simulink model "satellite_ADCS_slew_simulation"  (R2022b)
settings: Solver=FixedStepAuto  StartTime=t0  StopTime=t0+dt_po  FixedStep=0.1  RelTol=1e-9  AbsTol=1e-9
values from neighbouring files (symbols this model uses):
  A0 = Af    [satellite_ADCS_LEOP_simulation.m]
  A_sb_1 = [999.999999992226e-003    3.46376307675883e-006   -1.88420189887425e-006 ... (first row only)    [satellite_ADCS_LEOP_simulation.m]
  A_sb_2 = [999.999999948501e-003   -10.1488410044293e-006   -22.0178875132149e-012 ... (first row only)    [satellite_ADCS_LEOP_simulation.m]
  A_sb_3 = [999.999999975613e-003   -46.6812699606578e-012    6.98384920637069e-006 ... (first row only)    [satellite_ADCS_LEOP_simulation.m]
  alphaG_0 = pi/1.5    (= 2.09439510239)    [satellite_ADCS_LEOP_simulation.m]
  E = 1    [satellite_ADCS_LEOP_simulation.m]
  F = 1e-3    (= 0.001)    [satellite_ADCS_LEOP_simulation.m]
  FOV = deg2rad(21.7)    [satellite_ADCS_LEOP_simulation.m]
  g_nm = S_matrix.*g_coefficients    [satellite_ADCS_LEOP_simulation.m]
  h_nm = S_matrix.*h_coefficients    [satellite_ADCS_LEOP_simulation.m]
  J = diag([Ix,Iy,Iz])    [satellite_ADCS_LEOP_simulation.m]
  J2 = 1.082e-3    (= 0.001082)    [satellite_ADCS_LEOP_simulation.m]
  K_matrix = zeros(5,6)    [satellite_ADCS_LEOP_simulation.m]
  kdx = 0.001*450/8    (= 0.05625)    [satellite_ADCS_LEOP_simulation.m]
  kdy = kdx    (= 0.05625)    [satellite_ADCS_LEOP_simulation.m]
  kdz = kdy    (= 0.05625)    [satellite_ADCS_LEOP_simulation.m]
  kep = [a e i OM om thf]    [satellite_ADCS_LEOP_simulation.m]
  kpx = 0.6*0.001    (= 0.0006)    [satellite_ADCS_LEOP_simulation.m]
  kpy = kpx    (= 0.0006)    [satellite_ADCS_LEOP_simulation.m]
  kpz = kpy    (= 0.0006)    [satellite_ADCS_LEOP_simulation.m]
  LL = 1e-5    (= 1e-05)    [satellite_ADCS_LEOP_simulation.m]
  m = [0.37 0.32 0.28]    [satellite_ADCS_LEOP_simulation.m]
  mu = astroConstants(13)    [satellite_ADCS_LEOP_simulation.m]
  n_sun = 2*pi/T_y    (= 1.99238499086e-07)    [satellite_ADCS_LEOP_simulation.m]
  omega_e = 2*pi/T_e    (= 7.27220521664e-05)    [satellite_ADCS_LEOP_simulation.m]
  P00 = 1    [satellite_ADCS_LEOP_simulation.m]
  pR = pinv(R)    [satellite_ADCS_LEOP_simulation.m]
  R = [0 0 dz/2 0 0 -dz/2 ... (first row only)    [satellite_ADCS_LEOP_simulation.m]
  rt = astroConstants(23)    [satellite_ADCS_LEOP_simulation.m]
  S = S'    [satellite_ADCS_LEOP_simulation.m]
  sensor_noise = deg2rad(50/3600)    [satellite_ADCS_LEOP_simulation.m]
  sensor_sample_time = 1    [satellite_ADCS_LEOP_simulation.m]
  t0 = tf    (= 3200)    [satellite_ADCS_LEOP_simulation.m]
  T_o = 2*pi/n    [satellite_ADCS_LEOP_simulation.m]
  Te = 0.03    [satellite_ADCS_LEOP_simulation.m]
  Tp = [999.999926226686e-003    355.891478141766e-006   -144.526391847740e-006 ... (first row only)    [satellite_ADCS_LEOP_simulation.m]
  UL = 1e-4    (= 0.0001)    [satellite_ADCS_LEOP_simulation.m]
  w0 = wf    [satellite_ADCS_LEOP_simulation.m]
libraries: matrix_library x7, vrlib x3, slpidlib x3, sharedutil x2, aerolibutil x2
(part 3 of 3)

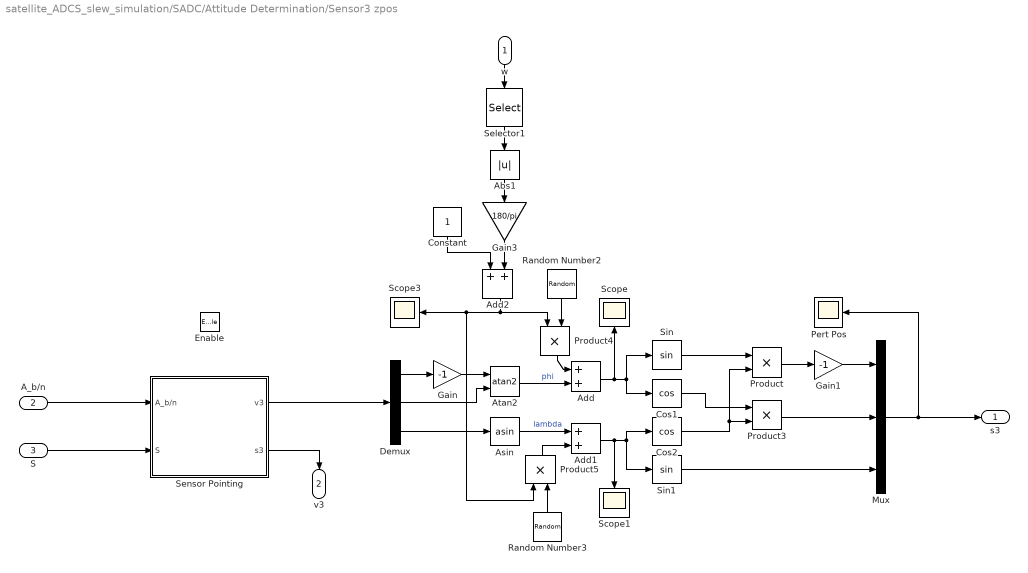
== system satellite_ADCS_slew_simulation/SADC/Attitude Determination/Sensor3 zpos ==
  w : Inport
  A_b/n : Inport  Port=2
  S : Inport  Port=3
  Enable : EnablePort  PropagateVarSize=During execution
  Abs1 : Abs  SaturateOnIntegerOverflow=off
  Add : Sum
  Add1 : Sum
  Add2 : Sum
  Asin : Trigonometry  Operator=asin
  Atan2 : Trigonometry  Operator=atan2
  Constant : Constant
  Cos1 : Trigonometry  Operator=cos
  Cos2 : Trigonometry  Operator=cos
  Demux : Demux  Outputs=3
  Gain : Gain  Gain=-1
  Gain1 : Gain  Gain=-1
  Gain3 : Gain  Gain=180/pi
  Mux : Mux  Inputs=3
  Pert Pos : Scope
  Product{,3..5} (4 alike) : Product
  Random Number2 : RandomNumber  Variance=sensor_noise^2  SampleTime=sensor_sample_time
  Random Number3 : RandomNumber  Variance=sensor_noise^2  SampleTime=sensor_sample_time
  Scope : Scope
  Scope1 : Scope
  Scope3 : Scope
  Selector1 : Selector  InputPortWidth=3  IndexOptions=Index vector (dialog)  Indices=3  OutputSizes=1
  Sensor Pointing : Subsystem
  Sin : Trigonometry
  Sin1 : Trigonometry
  s3 : Outport
  v3 : Outport  Port=2
  wires:
  Sensor Pointing/2(s3) -> v3/1
  Sensor Pointing/1(v3) -> Demux/1
  S/1 -> Sensor Pointing/2(S)
  A_b/n/1 -> Sensor Pointing/1(A_b/n)
  Gain1/1 -> Mux/1
  Sin1/1 -> Mux/3
  Mux/1 -> Pert Pos/1, s3/1
  Demux/3 -> Asin/1
  Product3/1 -> Mux/2
  Cos1/1 -> Product3/1
  Gain/1 -> Atan2/1
  Product/1 -> Gain1/1
  Sin/1 -> Product/1
  Add1/1 -> Cos2/1, Sin1/1, Scope1/1
  Cos2/1 -> Product3/2, Product/2
  Atan2/1 -> Add/2  "phi"
  Asin/1 -> Add1/1  "lambda"
  Demux/2 -> Atan2/2
  Add/1 -> Scope/1, Sin/1, Cos1/1
  Demux/1 -> Gain/1
  Product4/1 -> Add/1
  Product5/1 -> Add1/2
  w/1 -> Selector1/1
  Random Number2/1 -> Product4/2
  Add2/1 -> Product4/1, Scope3/1, Product5/1
  Selector1/1 -> Abs1/1
  Random Number3/1 -> Product5/2
  Abs1/1 -> Gain3/1
  Constant/1 -> Add2/1
  Gain3/1 -> Add2/2

== system satellite_ADCS_slew_simulation/SADC/Attitude Determination/Sun Sensors ==
  S_n : Inport
  A_b/n : Inport  Port=2
  Mux : Mux  Inputs=3
  Sun Sensor xpos : Subsystem
  Sun Sensor ypos : Subsystem
  Sun Sensor zpos : Subsystem
  Sun Obstruction : Outport
  wires:
  Mux/1 -> Sun Obstruction/1
  Sun Sensor zpos/1(s3) -> Mux/3
  Sun Sensor xpos/1(s1) -> Mux/1
  Sun Sensor ypos/1(s2) -> Mux/2
  S_n/1 -> Sun Sensor ypos/2(S_n), Sun Sensor zpos/2(S_n), Sun Sensor xpos/2(S_n)
  A_b/n/1 -> Sun Sensor ypos/1(A_b/n), Sun Sensor zpos/1(A_b/n), Sun Sensor xpos/1(A_b/n)

== system satellite_ADCS_slew_simulation/SADC/Attitude Determination/Wabha Attitude Determination ==
  s1 : Inport
  v1 : Inport  Port=2
  s2 : Inport  Port=3
  v2 : Inport  Port=4
  s3 : Inport  Port=5
  v3 : Inport  Port=6
  E : Inport  Port=7
  If : If  IfExpression=u1 == 3
  Merge : Merge
  Scope : Scope
  Sum of Elements : Sum  Inputs=+
  Wabha Attitude Determination 2s : Subsystem
  Wabha Attitude Determination 3s : Subsystem
  A*_b/n : Outport
  wires:
  v3/1 -> Wabha Attitude Determination 2s/7(v3), Wabha Attitude Determination 3s/6(v3)
  s3/1 -> Wabha Attitude Determination 2s/6(s3), Wabha Attitude Determination 3s/5(s3)
  v2/1 -> Wabha Attitude Determination 2s/5(v2), Wabha Attitude Determination 3s/4(v2)
  s2/1 -> Wabha Attitude Determination 2s/4(s2), Wabha Attitude Determination 3s/3(s2)
  v1/1 -> Wabha Attitude Determination 2s/3(v1), Wabha Attitude Determination 3s/2(v1)
  s1/1 -> Wabha Attitude Determination 2s/2(s1), Wabha Attitude Determination 3s/1(s1)
  Merge/1 -> A*_b/n/1
  If/1 -> Wabha Attitude Determination 3s/Action
  Wabha Attitude Determination 2s/1(A*_b/n) -> Merge/1
  If/2 -> Wabha Attitude Determination 2s/Action
  E/1 -> Sum of Elements/1, Wabha Attitude Determination 2s/1(E)
  Wabha Attitude Determination 3s/1(A*_b/n) -> Merge/2
  Sum of Elements/1 -> If/1, Scope/1

== system satellite_ADCS_slew_simulation/Euler Angles Kinematics/312 kin/R312/R1 ==
  a : Inport
  Add : Sum  Inputs=+++
  Constant : Constant  Value=[0 0 0; 0 1 0; 0 0 1]
  Constant1 : Constant  Value=[0 0 0; 0 0 -1; 0 1 0]
  Constant2 : Constant  Value=[1 0 0; 0 0 0; 0 0 0]
  Cos : Trigonometry  Operator=cos
  Product : Product
  Product1 : Product
  Sin : Trigonometry
  R1 : Outport
  wires:
  a/1 -> Cos/1, Sin/1
  Cos/1 -> Product/2
  Constant/1 -> Product/1
  Constant1/1 -> Product1/1
  Sin/1 -> Product1/2
  Product/1 -> Add/1
  Constant2/1 -> Add/3
  Product1/1 -> Add/2
  Add/1 -> R1/1

== system satellite_ADCS_slew_simulation/Euler Angles Kinematics/312 kin/R312/R2 ==
  a : Inport
  Add : Sum  Inputs=+++
  Constant : Constant  Value=[1 0 0; 0 0 0; 0 0 1]
  Constant1 : Constant  Value=[0 0 1; 0 0 0; -1 0 0]
  Constant2 : Constant  Value=[0 0 0; 0 1 0; 0 0 0]
  Cos : Trigonometry  Operator=cos
  Product : Product
  Product1 : Product
  Sin : Trigonometry
  R2 : Outport
  wires:
  a/1 -> Cos/1, Sin/1
  Cos/1 -> Product/2
  Constant/1 -> Product/1
  Constant1/1 -> Product1/1
  Sin/1 -> Product1/2
  Product/1 -> Add/1
  Constant2/1 -> Add/3
  Product1/1 -> Add/2
  Add/1 -> R2/1

== system satellite_ADCS_slew_simulation/Euler Angles Kinematics/312 kin/R312/R3 ==
  a : Inport
  Add : Sum  Inputs=+++
  Constant : Constant  Value=[1 0 0; 0 1 0; 0 0 0]
  Constant1 : Constant  Value=[0 -1 0; 1 0 0; 0 0 0]
  Constant2 : Constant  Value=[0 0 0; 0 0 0; 0 0 1]
  Cos : Trigonometry  Operator=cos
  Product : Product
  Product1 : Product
  Sin : Trigonometry
  R3 : Outport
  wires:
  a/1 -> Cos/1, Sin/1
  Cos/1 -> Product/2
  Constant/1 -> Product/1
  Constant1/1 -> Product1/1
  Sin/1 -> Product1/2
  Product/1 -> Add/1
  Constant2/1 -> Add/3
  Product1/1 -> Add/2
  Add/1 -> R3/1

== system satellite_ADCS_slew_simulation/Euler Angles Kinematics/312 kin/R313/R1 ==
  a : Inport
  Add : Sum  Inputs=+++
  Constant : Constant  Value=[0 0 0; 0 1 0; 0 0 1]
  Constant1 : Constant  Value=[0 0 0; 0 0 -1; 0 1 0]
  Constant2 : Constant  Value=[1 0 0; 0 0 0; 0 0 0]
  Cos : Trigonometry  Operator=cos
  Product : Product
  Product1 : Product
  Sin : Trigonometry
  R1 : Outport
  wires:
  a/1 -> Cos/1, Sin/1
  Cos/1 -> Product/2
  Constant/1 -> Product/1
  Constant1/1 -> Product1/1
  Sin/1 -> Product1/2
  Product/1 -> Add/1
  Constant2/1 -> Add/3
  Product1/1 -> Add/2
  Add/1 -> R1/1

== system satellite_ADCS_slew_simulation/Euler Angles Kinematics/312 kin/R313/R3 ==
  a : Inport
  Add : Sum  Inputs=+++
  Constant : Constant  Value=[1 0 0; 0 1 0; 0 0 0]
  Constant1 : Constant  Value=[0 -1 0; 1 0 0; 0 0 0]
  Constant2 : Constant  Value=[0 0 0; 0 0 0; 0 0 1]
  Cos : Trigonometry  Operator=cos
  Product : Product
  Product1 : Product
  Sin : Trigonometry
  R3 : Outport
  wires:
  a/1 -> Cos/1, Sin/1
  Cos/1 -> Product/2
  Constant/1 -> Product/1
  Constant1/1 -> Product1/1
  Sin/1 -> Product1/2
  Product/1 -> Add/1
  Constant2/1 -> Add/3
  Product1/1 -> Add/2
  Add/1 -> R3/1

== system satellite_ADCS_slew_simulation/Euler Angles Kinematics/312 kin/R313/R3' ==
  a : Inport
  Add : Sum  Inputs=+++
  Constant : Constant  Value=[1 0 0; 0 1 0; 0 0 0]
  Constant1 : Constant  Value=[0 -1 0; 1 0 0; 0 0 0]
  Constant2 : Constant  Value=[0 0 0; 0 0 0; 0 0 1]
  Cos : Trigonometry  Operator=cos
  Product : Product
  Product1 : Product
  Sin : Trigonometry
  R3 : Outport
  wires:
  a/1 -> Cos/1, Sin/1
  Cos/1 -> Product/2
  Constant/1 -> Product/1
  Constant1/1 -> Product1/1
  Sin/1 -> Product1/2
  Product/1 -> Add/1
  Constant2/1 -> Add/3
  Product1/1 -> Add/2
  Add/1 -> R3/1

== system satellite_ADCS_slew_simulation/Euler Angles Kinematics/313 kin/R312/R1 ==
  a : Inport
  Add : Sum  Inputs=+++
  Constant : Constant  Value=[0 0 0; 0 1 0; 0 0 1]
  Constant1 : Constant  Value=[0 0 0; 0 0 -1; 0 1 0]
  Constant2 : Constant  Value=[1 0 0; 0 0 0; 0 0 0]
  Cos : Trigonometry  Operator=cos
  Product : Product
  Product1 : Product
  Sin : Trigonometry
  R1 : Outport
  wires:
  a/1 -> Cos/1, Sin/1
  Cos/1 -> Product/2
  Constant/1 -> Product/1
  Constant1/1 -> Product1/1
  Sin/1 -> Product1/2
  Product/1 -> Add/1
  Constant2/1 -> Add/3
  Product1/1 -> Add/2
  Add/1 -> R1/1

== system satellite_ADCS_slew_simulation/Euler Angles Kinematics/313 kin/R312/R2 ==
  a : Inport
  Add : Sum  Inputs=+++
  Constant : Constant  Value=[1 0 0; 0 0 0; 0 0 1]
  Constant1 : Constant  Value=[0 0 1; 0 0 0; -1 0 0]
  Constant2 : Constant  Value=[0 0 0; 0 1 0; 0 0 0]
  Cos : Trigonometry  Operator=cos
  Product : Product
  Product1 : Product
  Sin : Trigonometry
  R2 : Outport
  wires:
  a/1 -> Cos/1, Sin/1
  Cos/1 -> Product/2
  Constant/1 -> Product/1
  Constant1/1 -> Product1/1
  Sin/1 -> Product1/2
  Product/1 -> Add/1
  Constant2/1 -> Add/3
  Product1/1 -> Add/2
  Add/1 -> R2/1

== system satellite_ADCS_slew_simulation/Euler Angles Kinematics/313 kin/R312/R3 ==
  a : Inport
  Add : Sum  Inputs=+++
  Constant : Constant  Value=[1 0 0; 0 1 0; 0 0 0]
  Constant1 : Constant  Value=[0 -1 0; 1 0 0; 0 0 0]
  Constant2 : Constant  Value=[0 0 0; 0 0 0; 0 0 1]
  Cos : Trigonometry  Operator=cos
  Product : Product
  Product1 : Product
  Sin : Trigonometry
  R3 : Outport
  wires:
  a/1 -> Cos/1, Sin/1
  Cos/1 -> Product/2
  Constant/1 -> Product/1
  Constant1/1 -> Product1/1
  Sin/1 -> Product1/2
  Product/1 -> Add/1
  Constant2/1 -> Add/3
  Product1/1 -> Add/2
  Add/1 -> R3/1

== system satellite_ADCS_slew_simulation/Euler Angles Kinematics/313 kin/R313/R1 ==
  a : Inport
  Add : Sum  Inputs=+++
  Constant : Constant  Value=[0 0 0; 0 1 0; 0 0 1]
  Constant1 : Constant  Value=[0 0 0; 0 0 -1; 0 1 0]
  Constant2 : Constant  Value=[1 0 0; 0 0 0; 0 0 0]
  Cos : Trigonometry  Operator=cos
  Product : Product
  Product1 : Product
  Sin : Trigonometry
  R1 : Outport
  wires:
  a/1 -> Cos/1, Sin/1
  Cos/1 -> Product/2
  Constant/1 -> Product/1
  Constant1/1 -> Product1/1
  Sin/1 -> Product1/2
  Product/1 -> Add/1
  Constant2/1 -> Add/3
  Product1/1 -> Add/2
  Add/1 -> R1/1

== system satellite_ADCS_slew_simulation/Euler Angles Kinematics/313 kin/R313/R3 ==
  a : Inport
  Add : Sum  Inputs=+++
  Constant : Constant  Value=[1 0 0; 0 1 0; 0 0 0]
  Constant1 : Constant  Value=[0 -1 0; 1 0 0; 0 0 0]
  Constant2 : Constant  Value=[0 0 0; 0 0 0; 0 0 1]
  Cos : Trigonometry  Operator=cos
  Product : Product
  Product1 : Product
  Sin : Trigonometry
  R3 : Outport
  wires:
  a/1 -> Cos/1, Sin/1
  Cos/1 -> Product/2
  Constant/1 -> Product/1
  Constant1/1 -> Product1/1
  Sin/1 -> Product1/2
  Product/1 -> Add/1
  Constant2/1 -> Add/3
  Product1/1 -> Add/2
  Add/1 -> R3/1

== system satellite_ADCS_slew_simulation/Euler Angles Kinematics/313 kin/R313/R3' ==
  a : Inport
  Add : Sum  Inputs=+++
  Constant : Constant  Value=[1 0 0; 0 1 0; 0 0 0]
  Constant1 : Constant  Value=[0 -1 0; 1 0 0; 0 0 0]
  Constant2 : Constant  Value=[0 0 0; 0 0 0; 0 0 1]
  Cos : Trigonometry  Operator=cos
  Product : Product
  Product1 : Product
  Sin : Trigonometry
  R3 : Outport
  wires:
  a/1 -> Cos/1, Sin/1
  Cos/1 -> Product/2
  Constant/1 -> Product/1
  Constant1/1 -> Product1/1
  Sin/1 -> Product1/2
  Product/1 -> Add/1
  Constant2/1 -> Add/3
  Product1/1 -> Add/2
  Add/1 -> R3/1

== system satellite_ADCS_slew_simulation/SADC/Attitude Determination/Algebraic Attitude Determination/2s Method ==
  S : Inport
  V : Inport  Port=2
  E : Inport  Port=3
  Enable : EnablePort  PropagateVarSize=During execution
  Cross Product{,1..3} (4 alike) : matrix_library/Cross Product
  Find Nonzero Elements : Find  NumberOfInputDimensions=3
  Invert 3x3 Matrix : aerolibutil/Invert  3x3 Matrix
  MatrixMultiply : Product  Multiplication=Matrix(*)
  Normalize Vector : vrlib/Utilities/Normalize Vector  maxzero=0
  Normalize Vector1 : vrlib/Utilities/Normalize Vector  maxzero=0
  Selector : Selector  NumberOfDimensions=2  InputPortWidth=3  IndexOptions=Index vector (dialog),Index vector (dialog)  Indices=[1 2 3],1  OutputSizes=1,1
  Selector1 : Selector  NumberOfDimensions=2  InputPortWidth=3  IndexOptions=Index vector (dialog),Index vector (dialog)  Indices=[1 2 3],2  OutputSizes=1,1
  Selector2 : Selector  NumberOfDimensions=2  InputPortWidth=3  IndexOptions=Index vector (dialog),Index vector (dialog)  Indices=[1 2 3],1  OutputSizes=1,1
  Selector3 : Selector  NumberOfDimensions=2  InputPortWidth=3  IndexOptions=Index vector (dialog),Index vector (dialog)  Indices=[1 2 3],2  OutputSizes=1,1
  Selector4 : Selector  NumberOfDimensions=2  InputPortWidth=3  IndexOptions=Index vector (dialog),Index vector (port)  Indices=[1 2 3],1  OutputSizes=1,1
  Selector5 : Selector  NumberOfDimensions=2  InputPortWidth=3  IndexOptions=Index vector (dialog),Index vector (port)  Indices=[1 2 3],1  OutputSizes=1,1
  Vector Concatenate : Concatenate  NumInputs=3  Mode=Multidimensional array  ConcatenateDimension=2
  Vector Concatenate1 : Concatenate  NumInputs=3  Mode=Multidimensional array  ConcatenateDimension=2
  A_b/n : Outport
  wires:
  S/1 -> Selector5/1  "S"
  V/1 -> Selector4/1  "V"
  Find Nonzero Elements/1 -> Selector4/2, Selector5/2
  E/1 -> Find Nonzero Elements/1
  MatrixMultiply/1 -> A_b/n/1
  Invert 3x3 Matrix/1 -> MatrixMultiply/2
  Vector Concatenate1/1 -> Invert 3x3 Matrix/1  "V"
  Vector Concatenate/1 -> MatrixMultiply/1  "S"
  Cross Product3/1 -> Vector Concatenate1/3
  Cross Product2/1 -> Vector Concatenate/3
  Normalize Vector/1 -> Cross Product3/2, Vector Concatenate1/2
  Normalize Vector1/1 -> Cross Product2/2, Vector Concatenate/2
  Cross Product/1 -> Normalize Vector1/1
  Cross Product1/1 -> Normalize Vector/1
  Selector3/1 -> Cross Product1/2  "b"
  Selector2/1 -> Cross Product1/1, Vector Concatenate1/1, Cross Product3/1  "a"
  Selector1/1 -> Cross Product/2  "q"
  Selector/1 -> Cross Product2/1, Vector Concatenate/1, Cross Product/1  "p"
  Selector5/1 -> Selector/1, Selector1/1  "S"
  Selector4/1 -> Selector2/1, Selector3/1  "V"

== system satellite_ADCS_slew_simulation/SADC/Attitude Determination/Algebraic Attitude Determination/3s Method ==
  S : Inport
  V : Inport  Port=2
  Enable : EnablePort  PropagateVarSize=During execution
  Invert 3x3 Matrix1 : aerolibutil/Invert  3x3 Matrix
  MatrixMultiply3 : Product  Multiplication=Matrix(*)
  A_b/n : Outport
  wires:
  S/1 -> MatrixMultiply3/1  "S"
  Invert 3x3 Matrix1/1 -> MatrixMultiply3/2  "V*"
  MatrixMultiply3/1 -> A_b/n/1
  V/1 -> Invert 3x3 Matrix1/1  "V"

== system satellite_ADCS_slew_simulation/SADC/Attitude Determination/Sensor1 xpos/Sensor Pointing ==
  note: A_b/n is already discretized
  note: A_sb is relative to the sensor
  note: star catalogue in inertial frame
  A_b/n : Inport
  S : Inport  Port=2
  . : Product  Multiplication=Matrix(*)
  Constant2 : Constant  Value=A_sb_1
  Constant4 : Constant  Value=FOV/2
  Cos : Trigonometry  Operator=cos
  Find Nonzero Elements1 : Find  NumberOfInputDimensions=3
  Less Than1 : RelationalOperator  OutDataTypeStr=boolean  RndMeth=Simplest  InputSameDT=off
  MinMax2 : MinMax
  Product1 : Product  Multiplication=Matrix(*)
  Scope3 : Scope
  Selector1 : Selector  NumberOfDimensions=2  InputPortWidth=3  IndexOptions=Index vector (dialog),Index vector (port)  Indices=[1 2 3],1  OutputSizes=1,1
  Selector2 : Selector  NumberOfDimensions=2  InputPortWidth=3  IndexOptions=Index vector (dialog),Index vector (port)  Indices=[1 2 3],1  OutputSizes=1,1
  x : Selector  NumberOfDimensions=2  InputPortWidth=3  IndexOptions=Index vector (dialog),Index vector (dialog)  Indices=1,1:162  OutputSizes=1,1
  s1 : Outport
  v1 : Outport  Port=2
  wires:
  A_b/n/1 -> Product1/2
  Selector1/1 -> v1/1
  Less Than1/1 -> Find Nonzero Elements1/1
  Cos/1 -> Less Than1/2
  x/1 -> Less Than1/1
  Product1/1 -> ./1  "A_s/n"
  S/1 -> ./2, Selector1/1
  Find Nonzero Elements1/1 -> MinMax2/1
  Constant4/1 -> Cos/1
  ./1 -> x/1, Selector2/1
  Selector2/1 -> Scope3/1, s1/1
  Constant2/1 -> Product1/1
  MinMax2/1 -> Selector1/2, Selector2/2

== system satellite_ADCS_slew_simulation/SADC/Attitude Determination/Sensor2 ypos/Sensor Pointing ==
  note: star catalogue in inertial frame
  note: A_sb is relative to the sensor
  note: A_b/n is already discretized
  A_b/n : Inport
  S : Inport  Port=2
  . : Product  Multiplication=Matrix(*)
  Constant2 : Constant  Value=A_sb_2
  Constant4 : Constant  Value=FOV/2
  Cos : Trigonometry  Operator=cos
  Find Nonzero Elements1 : Find  NumberOfInputDimensions=3
  Less Than1 : RelationalOperator  OutDataTypeStr=boolean  RndMeth=Simplest  InputSameDT=off
  MinMax2 : MinMax
  Product1 : Product  Multiplication=Matrix(*)
  Scope3 : Scope
  Selector1 : Selector  NumberOfDimensions=2  InputPortWidth=3  IndexOptions=Index vector (dialog),Index vector (port)  Indices=[1 2 3],1  OutputSizes=1,1
  Selector2 : Selector  NumberOfDimensions=2  InputPortWidth=3  IndexOptions=Index vector (dialog),Index vector (port)  Indices=[1 2 3],1  OutputSizes=1,1
  y : Selector  NumberOfDimensions=2  InputPortWidth=3  IndexOptions=Index vector (dialog),Index vector (dialog)  Indices=2,1:162  OutputSizes=1,1
  s2 : Outport
  v2 : Outport  Port=2
  wires:
  A_b/n/1 -> Product1/2
  Selector1/1 -> v2/1
  S/1 -> Selector1/1, ./2
  ./1 -> Selector2/1, y/1
  Constant4/1 -> Cos/1
  y/1 -> Less Than1/1
  Product1/1 -> ./1  "A_s/n"
  Find Nonzero Elements1/1 -> MinMax2/1
  Cos/1 -> Less Than1/2
  Constant2/1 -> Product1/1
  MinMax2/1 -> Selector2/2, Selector1/2
  Selector2/1 -> Scope3/1, s2/1
  Less Than1/1 -> Find Nonzero Elements1/1

== system satellite_ADCS_slew_simulation/SADC/Attitude Determination/Sensor3 zpos/Sensor Pointing ==
  note: A_b/n is already discretized
  note: A_sb is relative to the sensor
  note: star catalogue in inertial frame
  A_b/n : Inport
  S : Inport  Port=2
  . : Product  Multiplication=Matrix(*)
  Constant2 : Constant  Value=A_sb_3
  Constant4 : Constant  Value=FOV/2
  Cos : Trigonometry  Operator=cos
  Find Nonzero Elements1 : Find  NumberOfInputDimensions=3
  Less Than1 : RelationalOperator  OutDataTypeStr=boolean  RndMeth=Simplest  InputSameDT=off
  MinMax2 : MinMax
  Product1 : Product  Multiplication=Matrix(*)
  Scope3 : Scope
  Selector1 : Selector  NumberOfDimensions=2  InputPortWidth=3  IndexOptions=Index vector (dialog),Index vector (port)  Indices=[1 2 3],1  OutputSizes=1,1
  Selector2 : Selector  NumberOfDimensions=2  InputPortWidth=3  IndexOptions=Index vector (dialog),Index vector (port)  Indices=[1 2 3],1  OutputSizes=1,1
  z : Selector  NumberOfDimensions=2  InputPortWidth=3  IndexOptions=Index vector (dialog),Index vector (dialog)  Indices=3,1:162  OutputSizes=1,1
  v3 : Outport
  s3 : Outport  Port=2
  wires:
  Selector1/1 -> s3/1
  Product1/1 -> ./1  "A_s/n"
  z/1 -> Less Than1/1
  A_b/n/1 -> Product1/2
  Constant2/1 -> Product1/1
  Cos/1 -> Less Than1/2
  Less Than1/1 -> Find Nonzero Elements1/1
  ./1 -> z/1, Selector2/1
  S/1 -> ./2, Selector1/1
  Selector2/1 -> Scope3/1, v3/1
  MinMax2/1 -> Selector1/2, Selector2/2
  Constant4/1 -> Cos/1
  Find Nonzero Elements1/1 -> MinMax2/1

== system satellite_ADCS_slew_simulation/SADC/Attitude Determination/Sun Sensors/Sun Sensor xpos ==
  note: A_sb is relative to the sensor
  A_b/n : Inport
  S_n : Inport  Port=2
  . : Product  Multiplication=Matrix(*)
  Constant2 : Constant  Value=A_sb_1
  Constant4 : Constant  Value=1.5*FOV/2
  Cos : Trigonometry  Operator=cos
  Less Than1 : RelationalOperator  Operator=<=  OutDataTypeStr=boolean  RndMeth=Simplest  InputSameDT=off
  Product1 : Product  Multiplication=Matrix(*)
  x : Selector  InputPortWidth=3  IndexOptions=Index vector (dialog)  Indices=1  OutputSizes=1
  s1 : Outport
  wires:
  A_b/n/1 -> Product1/2
  Cos/1 -> Less Than1/2
  x/1 -> Less Than1/1
  Product1/1 -> ./1  "A_s/n"
  S_n/1 -> ./2
  Constant4/1 -> Cos/1
  ./1 -> x/1
  Less Than1/1 -> s1/1
  Constant2/1 -> Product1/1

== system satellite_ADCS_slew_simulation/SADC/Attitude Determination/Sun Sensors/Sun Sensor ypos ==
  note: A_sb is relative to the sensor
  A_b/n : Inport
  S_n : Inport  Port=2
  . : Product  Multiplication=Matrix(*)
  Constant2 : Constant  Value=A_sb_2
  Constant4 : Constant  Value=1.5*FOV/2
  Cos : Trigonometry  Operator=cos
  Less Than1 : RelationalOperator  Operator=<=  OutDataTypeStr=boolean  RndMeth=Simplest  InputSameDT=off
  Product1 : Product  Multiplication=Matrix(*)
  y : Selector  InputPortWidth=3  IndexOptions=Index vector (dialog)  Indices=2  OutputSizes=1
  s2 : Outport
  wires:
  A_b/n/1 -> Product1/2
  S_n/1 -> ./2
  ./1 -> y/1
  Constant4/1 -> Cos/1
  y/1 -> Less Than1/1
  Product1/1 -> ./1  "A_s/n"
  Cos/1 -> Less Than1/2
  Constant2/1 -> Product1/1
  Less Than1/1 -> s2/1

== system satellite_ADCS_slew_simulation/SADC/Attitude Determination/Sun Sensors/Sun Sensor zpos ==
  note: A_sb is relative to the sensor
  A_b/n : Inport
  S_n : Inport  Port=2
  . : Product  Multiplication=Matrix(*)
  Constant2 : Constant  Value=A_sb_3
  Constant4 : Constant  Value=1.5*FOV/2
  Cos : Trigonometry  Operator=cos
  Less Than1 : RelationalOperator  Operator=<=  OutDataTypeStr=boolean  RndMeth=Simplest  InputSameDT=off
  Product1 : Product  Multiplication=Matrix(*)
  z : Selector  InputPortWidth=3  IndexOptions=Index vector (dialog)  Indices=3  OutputSizes=1
  s3 : Outport
  wires:
  Product1/1 -> ./1  "A_s/n"
  z/1 -> Less Than1/1
  A_b/n/1 -> Product1/2
  Constant2/1 -> Product1/1
  Cos/1 -> Less Than1/2
  Less Than1/1 -> s3/1
  ./1 -> z/1
  S_n/1 -> ./2
  Constant4/1 -> Cos/1

== system satellite_ADCS_slew_simulation/SADC/Attitude Determination/Wabha Attitude Determination/Wabha Attitude Determination 2s ==
  E : Inport
  s1 : Inport  Port=2
  v1 : Inport  Port=3
  s2 : Inport  Port=4
  v2 : Inport  Port=5
  s3 : Inport  Port=6
  v3 : Inport  Port=7
  Action Port : ActionPort  PropagateVarSize=During execution  ActionPortLabel=else
  Add : Sum
  Constant3 : Constant  Value=1/2
  Find Nonzero Elements : Find  NumberOfInputDimensions=3
  MATLAB Function : MATLAB Function  TreatAsAtomicUnit=on
  Product : Product
  Product1 : Product
  Product3 : Product  Multiplication=Matrix(*)
  Product4 : Product  Multiplication=Matrix(*)
  Selector : Selector  NumberOfDimensions=2  InputPortWidth=3  IndexOptions=Index vector (dialog),Index vector (port)  Indices=[1 2 3],1  OutputSizes=1,1
  Selector1 : Selector  NumberOfDimensions=2  InputPortWidth=3  IndexOptions=Index vector (dialog),Index vector (port)  Indices=[1 2 3],1  OutputSizes=1,1
  Selector2 : Selector  NumberOfDimensions=2  InputPortWidth=3  IndexOptions=Index vector (dialog),Index vector (dialog)  Indices=[1 2 3],1  OutputSizes=1,1
  Selector3 : Selector  NumberOfDimensions=2  InputPortWidth=3  IndexOptions=Index vector (dialog),Index vector (dialog)  Indices=[1 2 3],2  OutputSizes=1,1
  Selector4 : Selector  NumberOfDimensions=2  InputPortWidth=3  IndexOptions=Index vector (dialog),Index vector (dialog)  Indices=[1 2 3],1  OutputSizes=1,1
  Selector5 : Selector  NumberOfDimensions=2  InputPortWidth=3  IndexOptions=Index vector (dialog),Index vector (dialog)  Indices=[1 2 3],2  OutputSizes=1,1
  Transpose : Math  Operator=transpose
  Transpose1 : Math  Operator=transpose
  Vector Concatenate : Concatenate  NumInputs=3  Mode=Multidimensional array  ConcatenateDimension=2
  Vector Concatenate1 : Concatenate  NumInputs=3  Mode=Multidimensional array  ConcatenateDimension=2
  A*_b/n : Outport
  wires:
  Constant3/1 -> Product/2, Product1/2
  MATLAB Function/1(y) -> A*_b/n/1
  Product1/1 -> Add/2
  Product/1 -> Add/1
  Transpose1/1 -> Product4/2
  Transpose/1 -> Product3/2
  Selector5/1 -> Transpose1/1  "v2"
  Selector4/1 -> Transpose/1  "v1"
  Selector3/1 -> Product4/1  "s2"
  Selector2/1 -> Product3/1  "s1"
  Product4/1 -> Product1/1
  Product3/1 -> Product/1
  Add/1 -> MATLAB Function/1(u)
  Selector/1 -> Selector5/1, Selector4/1
  Selector1/1 -> Selector2/1, Selector3/1
  Find Nonzero Elements/1 -> Selector1/2, Selector/2
  Vector Concatenate/1 -> Selector1/1
  Vector Concatenate1/1 -> Selector/1
  E/1 -> Find Nonzero Elements/1
  v1/1 -> Vector Concatenate1/1
  v2/1 -> Vector Concatenate1/2
  v3/1 -> Vector Concatenate1/3
  s3/1 -> Vector Concatenate/3
  s2/1 -> Vector Concatenate/2
  s1/1 -> Vector Concatenate/1

== system satellite_ADCS_slew_simulation/SADC/Attitude Determination/Wabha Attitude Determination/Wabha Attitude Determination 3s ==
  s1 : Inport
  v1 : Inport  Port=2
  s2 : Inport  Port=3
  v2 : Inport  Port=4
  s3 : Inport  Port=5
  v3 : Inport  Port=6
  Action Port : ActionPort  PropagateVarSize=During execution  ActionPortLabel=if(u1 == 3)
  Constant3 : Constant  Value=1/3
  MATLAB Function : MATLAB Function  TreatAsAtomicUnit=on
  Product : Product  Multiplication=Matrix(*)
  Product1 : Product  Multiplication=Matrix(*)
  Product2 : Product  Multiplication=Matrix(*)
  Product3 : Product
  Product4 : Product
  Product5 : Product
  Sum : Sum  Inputs=+++
  Transpose : Math  Operator=transpose
  Transpose1 : Math  Operator=transpose
  Transpose2 : Math  Operator=transpose
  A*_b/n : Outport
  wires:
  Constant3/1 -> Product5/2, Product4/2, Product3/2
  Sum/1 -> MATLAB Function/1(u)  "B"
  MATLAB Function/1(y) -> A*_b/n/1
  v1/1 -> Transpose/1
  Product5/1 -> Sum/3
  Product3/1 -> Sum/1
  Product4/1 -> Sum/2
  Product2/1 -> Product5/1
  Product1/1 -> Product4/1
  Product/1 -> Product3/1
  Transpose2/1 -> Product2/2
  s3/1 -> Product2/1
  s2/1 -> Product1/1
  Transpose1/1 -> Product1/2
  Transpose/1 -> Product/2
  s1/1 -> Product/1
  v3/1 -> Transpose2/1
  v2/1 -> Transpose1/1

== matlab function satellite_ADCS_slew_simulation/SADC/Attitude Determination/Wabha Attitude Determination/Wabha Attitude Determination 3s/MATLAB Function ==
  data: u input; y output
function y  = fun(u)
[U,S,V] = svd(u);
M = diag([1 1 det(U)*det(V)]);
y = U*(M*(V'));
end

== matlab function satellite_ADCS_slew_simulation/SADC/Attitude Determination/Wabha Attitude Determination/Wabha Attitude Determination 2s/MATLAB Function ==
  data: u input; y output
function y  = fun(u)
[U,S,V] = svd(u);
M = diag([1 1 det(U)*det(V)]);
y = U*(M*(V'));
end
